simulink model "q19a"  (R2016a)
settings: Solver=VariableStepAuto  StartTime=0.0  StopTime=10.0  RelTol=1e-3
settings Model: Creator=Satya  LastModifiedBy=Satya

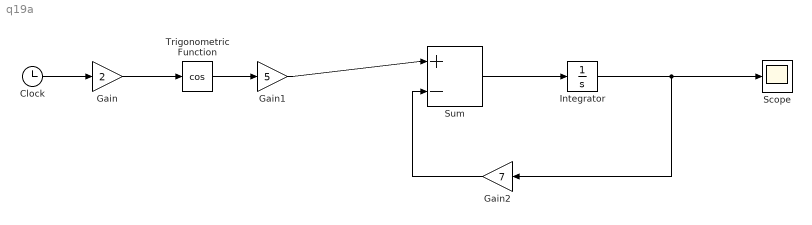
== system q19a ==
  Clock : Clock
  Gain : Gain  Gain=2
  Gain1 : Gain  Gain=5
  Gain2 : Gain  Gain=7
  Integrator : Integrator
  Scope : Scope
  Sum : Sum  Inputs=|+-
  Trigonometric Function : Trigonometry  Operator=cos
  wires:
  Trigonometric Function/1 -> Gain1/1
  Sum/1 -> Integrator/1
  Integrator/1 -> Gain2/1, Scope/1
  Gain1/1 -> Sum/1
  Gain/1 -> Trigonometric Function/1
  Clock/1 -> Gain/1
  Gain2/1 -> Sum/2
